simulink model "environment_service"  (R2026a)
settings: Solver=VariableStepAuto  StopTime=10
settings Model: Creator=asus  LastModifiedBy=asus

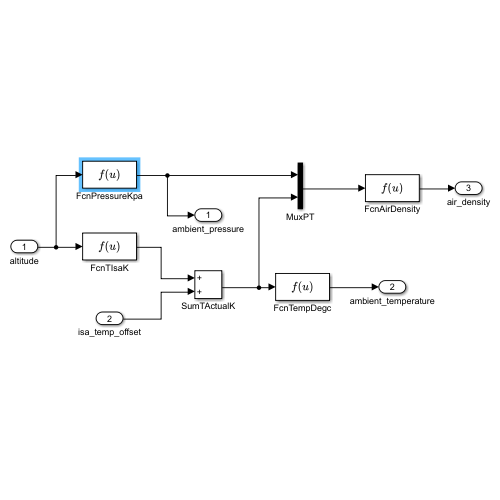
[thumbnail: Simulink's stored preview of the top-level diagram]
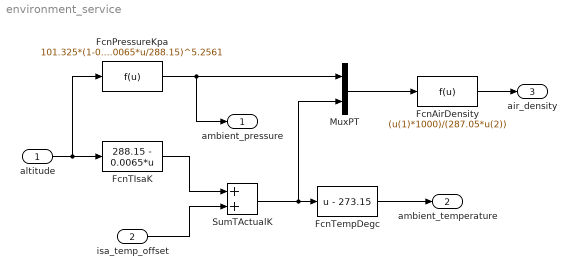
== system environment_service ==
  altitude : Inport
  isa_temp_offset : Inport  Port=2
  FcnAirDensity : Fcn  Expr=(u(1)*1000)/(287.05*u(2))
  FcnPressureKpa : Fcn  Expr=101.325*(1-0.0065*u/288.15)^5.2561
  FcnTIsaK : Fcn  Expr=288.15 - 0.0065*u
  FcnTempDegc : Fcn  Expr=u - 273.15
  MuxPT : Mux  Inputs=2
  SumTActualK : Sum
  ambient_pressure : Outport
  ambient_temperature : Outport  Port=2
  air_density : Outport  Port=3
  wires:
  altitude/1 -> FcnPressureKpa/1, FcnTIsaK/1
  FcnTIsaK/1 -> SumTActualK/1
  isa_temp_offset/1 -> SumTActualK/2
  SumTActualK/1 -> MuxPT/2, FcnTempDegc/1
  FcnPressureKpa/1 -> MuxPT/1, ambient_pressure/1
  MuxPT/1 -> FcnAirDensity/1
  FcnTempDegc/1 -> ambient_temperature/1
  FcnAirDensity/1 -> air_density/1
